simulink model "EV_ControlSystem_Architecture_Harness1"  (R2025b)
settings: Solver=FixedStepAuto  StartTime=0.0  StopTime=40  FixedStep=0.1  RelTol=1e-3
undefined symbols (not defined in the file or in its folder): SOCInit
libraries: SignalEditorBlockLib x2
(part 1 of 3)
settings Model: DataDictionary=systemParams.sldd  PacingRate=3  Creator=smuckati  LastModifiedBy=smuckati
settings OptimizationCC: UseDivisionForNetSlopeComputation=on
settings DebuggingCC: ParameterPrecisionLossMsg=none
settings ModelReferenceCC: ModelReferenceNumInstancesAllowed=Single
settings RTWCC: GPUComputeCapability=3.5
settings GRTTargetCC: SubcomponentCodeInterfacePackaging=Nonreusable function

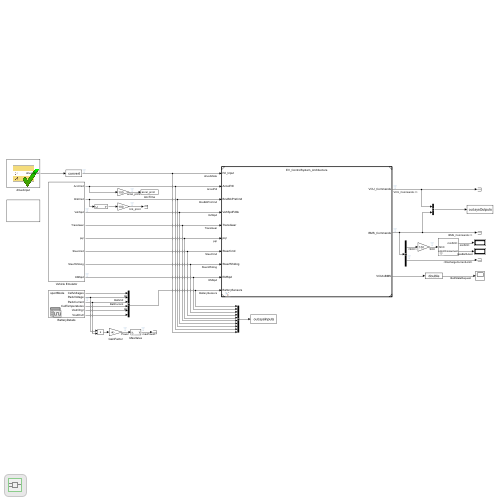
[thumbnail: Simulink's stored preview of the top-level diagram]
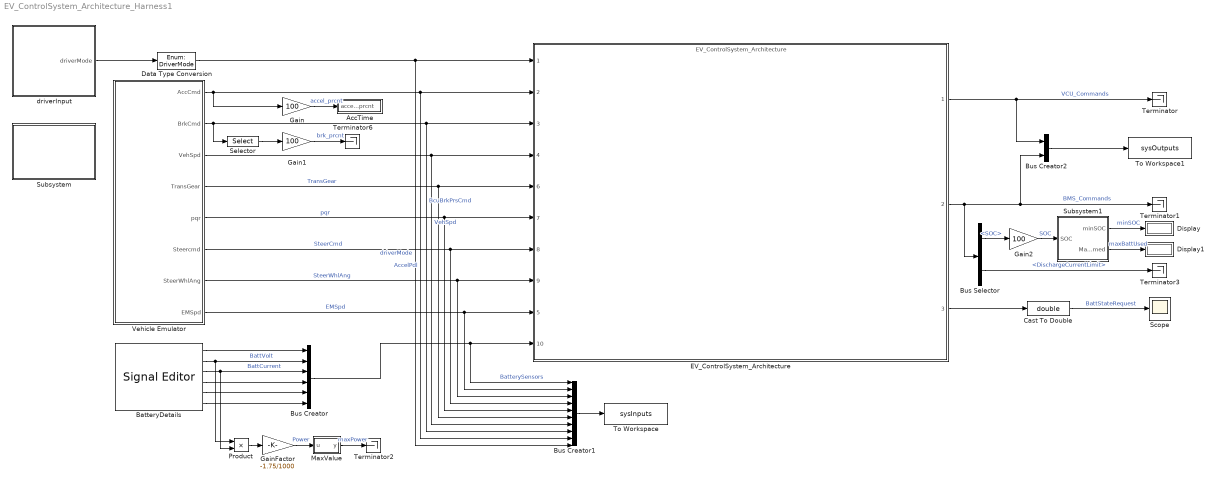
== system EV_ControlSystem_Architecture_Harness1 ==
  AccTime : Subsystem
  BatteryDetails : SignalEditorBlockLib/Signal Editor  FileName=BMSInputs.mat  ActiveScenario=sportMode  ActiveSignal=CellVoltages  IsBus=off  OutputBusObjectStr=Bus: BusObject  SampleTime=0  Interpolate=off  ZeroCross=off  OutputAfterFinalValue=Setting to zero  Unit=inherit  PreserveSignalName=on  ApplySigPropsToAllScenarios=on  ApplySigPropsToAllSignals=off  SignalPropertySource=Dialog parameters
  Bus Creator : BusCreator  Inputs=6  OutDataTypeStr=Bus: Sensors
      settings: InheritFromInputs=off
  Bus Creator1 : BusCreator  Inputs=10
  Bus Creator2 : BusCreator  Inputs=2
  Bus Selector : BusSelector  OutputSignals=SOC,CurrentLimits.DischargeCurrentLimit
  Cast To Double : DataTypeConversion  OutDataTypeStr=double  SaturateOnIntegerOverflow=off  RndMeth=Floor
  Data Type Conversion : DataTypeConversion  OutDataTypeStr=Enum: DriverMode  SaturateOnIntegerOverflow=off  RndMeth=Floor
  Display : Display
  Display1 : Display
  EV_ControlSystem_Architecture : ModelReference  ModelNameDialog=EV_ControlSystem_Architecture  SimulationMode=Normal  ModelReferenceVersion=6.0
      settings: PortSchema="{\"entries\":[{\"content\":{\"sides\":[{\"content\":{\"connectorIds\":[\"In1\",\"In2\",\"In3\",\"In4\",\"In6\",\"In7\",\"In8\",\"In9\",\"In5\",\"In10\"]},\"type\":\"ConnectorPlacement.EquallySpacedRectSide\",\"uuid\":\"aec7a944-4e11-4ff9-b38b-241836784c73\"},{\"content\":{\"connectorIds\":[\"Out1\",\"Out2\",\"Out3\"],\"side\":\"RIGHT\"},\"type\":\"ConnectorPlacement.EquallySpacedRectSide\",\"uuid\":\"2d27f022-c07c-42c9-8c83-6c3bf1c857c3\"},{\"content\":{\"side\":\"TOP\"},\"type\":\"ConnectorPlacement.EquallySpacedRectSide\",\"uuid\":\"0fd9c3f7-3419-4d87-af59-340823930bd8\"}]},\"type\":\"ConnectorPlacement.EquallySpacedConnector\",\"uuid\":\"96ad767e-9848-423d-9456-8b436e831e2a\"}],\"packageUris\":[\"http://schema.mathworks.com/mf0/Connector/R2020b\"],\"version\":\"1.0\"}"
  Gain : Gain  Gain=100
  Gain1 : Gain  Gain=100
  Gain2 : Gain  Gain=100
  GainFactor : Gain  Gain=-1.75/1000
  MaxValue : Subsystem  mask{initVal=0}
      mask prompts: initVal "Init SOC Value"
  Product : Product
  Scope : Scope
  Selector : Selector  InputPortWidth=4  IndexOptions=Index vector (dialog)  Indices=[1]  OutputSizes=1
  Subsystem : Subsystem
  Subsystem1 : Subsystem  mask{initVal=SOCInit}
      mask prompts: initVal "Init SOC Value"
  Terminator{,1..3,6} (5 alike) : Terminator
  To Workspace : ToWorkspace  VariableName=sysInputs  SaveFormat=Timeseries  SampleTime=-1
  To Workspace1 : ToWorkspace  VariableName=sysOutputs  SaveFormat=Timeseries  SampleTime=-1
  Vehicle Emulator : Subsystem
  driverInput : Test Sequence  TreatAsAtomicUnit=on
  wires:
  BatteryDetails/6 -> Bus Creator/6
  BatteryDetails/5 -> Bus Creator/5
  BatteryDetails/4 -> Bus Creator/4
  BatteryDetails/3 -> Product/2, Bus Creator/3  "BattCurrent"
  BatteryDetails/2 -> Bus Creator/2, Product/1  "BattVolt"
  BatteryDetails/1 -> Bus Creator/1
  Data Type Conversion/1 -> Bus Creator1/10, EV_ControlSystem_Architecture/1  "driverMode"
  Vehicle Emulator/1(AccCmd) -> Gain/1, Bus Creator1/9, EV_ControlSystem_Architecture/2  "AccelPdl"
  Vehicle Emulator/2(BrkCmd) -> Selector/1, Bus Creator1/8, EV_ControlSystem_Architecture/3  "BcuBrkPrsCmd"
  Vehicle Emulator/3(VehSpd) -> Bus Creator1/7, EV_ControlSystem_Architecture/4  "VehSpd"
  Vehicle Emulator/8(EMSpd) -> Bus Creator1/2, EV_ControlSystem_Architecture/5  "EMSpd"
  Vehicle Emulator/4(TransGear) -> Bus Creator1/6, EV_ControlSystem_Architecture/6  "TransGear"
  Vehicle Emulator/5(pqr) -> Bus Creator1/5, EV_ControlSystem_Architecture/7  "pqr"
  Vehicle Emulator/6(Steercmd) -> Bus Creator1/4, EV_ControlSystem_Architecture/8  "SteerCmd"
  Vehicle Emulator/7(SteerWhlAng) -> Bus Creator1/3, EV_ControlSystem_Architecture/9  "SteerWhlAng"
  EV_ControlSystem_Architecture/1 -> Bus Creator2/1, Terminator/1  "VCU_Commands"
  EV_ControlSystem_Architecture/2 -> Bus Selector/1, Bus Creator2/2, Terminator1/1  "BMS_Commands"
  Bus Selector/2 -> Terminator3/1  "<DischargeCurrentLimit>"
  Bus Selector/1 -> Gain2/1  "<SOC>"
  Gain/1 -> AccTime/1(accel_prcnt)  "accel_prcnt"
  Gain1/1 -> Terminator6/1  "brk_prcnt"
  Bus Creator/1 -> Bus Creator1/1, EV_ControlSystem_Architecture/10  "BatterySensors"
  Selector/1 -> Gain1/1
  driverInput/1(driverMode) -> Data Type Conversion/1
  Gain2/1 -> Subsystem1/1(SOC)  "SOC"
  Subsystem1/1(minSOC) -> Display/1  "minSOC"
  Bus Creator1/1 -> To Workspace/1
  Bus Creator2/1 -> To Workspace1/1
  Subsystem1/2(MaxBattConsumed) -> Display1/1  "maxBattUsed"
  EV_ControlSystem_Architecture/3 -> Cast To Double/1
  Cast To Double/1 -> Scope/1  "BattStateRequest"
  Product/1 -> GainFactor/1
  GainFactor/1 -> MaxValue/1(u)  "Power"
  MaxValue/1(y) -> Terminator2/1  "maxPower"

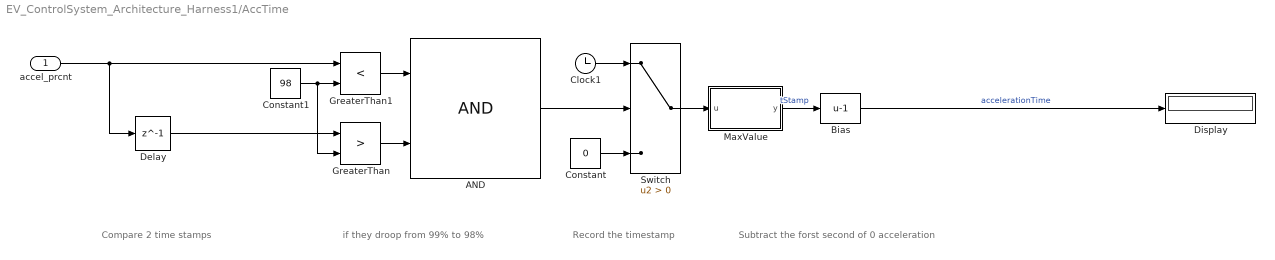
== system EV_ControlSystem_Architecture_Harness1/AccTime ==
  note: Compare 2 time stamps
  note: if they droop from 99% to 98%
  note: Record the timestamp
  note: Subtract the forst second of 0 acceleration
  accel_prcnt : Inport
  AND : Logic  IconShape=distinctive  AllPortsSameDT=off  OutDataTypeStr=boolean
  Bias : Bias  Bias=-1  SaturateOnIntegerOverflow=off
  Clock1 : Clock
  Constant : Constant  Value=0
  Constant1 : Constant  Value=98
  Delay : Delay  DelayLength=1
  Display : Display
  GreaterThan : RelationalOperator  Operator=>  OutDataTypeStr=boolean  RndMeth=Simplest  InputSameDT=off
  GreaterThan1 : RelationalOperator  Operator=<  OutDataTypeStr=boolean  RndMeth=Simplest  InputSameDT=off
  MaxValue : Subsystem  mask{initVal=0}
      mask prompts: initVal "Init SOC Value"
  Switch : Switch  Criteria=u2 > Threshold  SaturateOnIntegerOverflow=off  InputSameDT=off
  wires:
  Constant1/1 -> GreaterThan/2, GreaterThan1/2
  Constant/1 -> Switch/3
  AND/1 -> Switch/2
  accel_prcnt/1 -> Delay/1, GreaterThan1/1
  GreaterThan1/1 -> AND/1
  Delay/1 -> GreaterThan/1
  Switch/1 -> MaxValue/1(u)
  MaxValue/1(y) -> Bias/1  "tStamp"
  GreaterThan/1 -> AND/2
  Bias/1 -> Display/1  "accelerationTime"
  Clock1/1 -> Switch/1

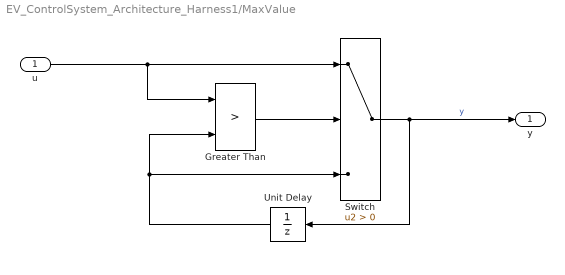
== system EV_ControlSystem_Architecture_Harness1/MaxValue ==
  u : Inport
  Greater Than : RelationalOperator  Operator=>  OutDataTypeStr=boolean  RndMeth=Simplest  InputSameDT=off
  Switch : Switch  Criteria=u2 > Threshold  SaturateOnIntegerOverflow=off  InputSameDT=off
  Unit Delay : UnitDelay  SampleTime=-1  HasFrameUpgradeWarning=on
  y : Outport
  wires:
  u/1 -> Switch/1, Greater Than/1
  Unit Delay/1 -> Greater Than/2, Switch/3
  Switch/1 -> Unit Delay/1, y/1  "y"
  Greater Than/1 -> Switch/2
